simulink model "NavFilterTestHarness24"  (R2024b)
settings: Solver=FixedStepDiscrete  StartTime=startTime  StopTime=endTime  FixedStep=0.001  RelTol=1e-3  EnableMultiTasking=on
undefined symbols (not defined in the file): accel, ADSframe, ADStime, alignTime, angRate, ATTframe, CourseDeg, EAS2TAS, GndSpd, GPSframe, GPStime, Hgt, IMUframe, IMUtime, LatDeg, LngDeg, MagBiasX, MagBiasY, MagBiasZ, MAGframe, MAGtime, MagX, MagY, MagZ, msecHgtDelay, msecMagDelay, msecPosDelay, msecTasDelay, msecVelDelay, Pitch, Roll, Veas, VelD, Yaw
libraries: simulink x9, simulink_need_slupdate x2
(part 2 of 5)

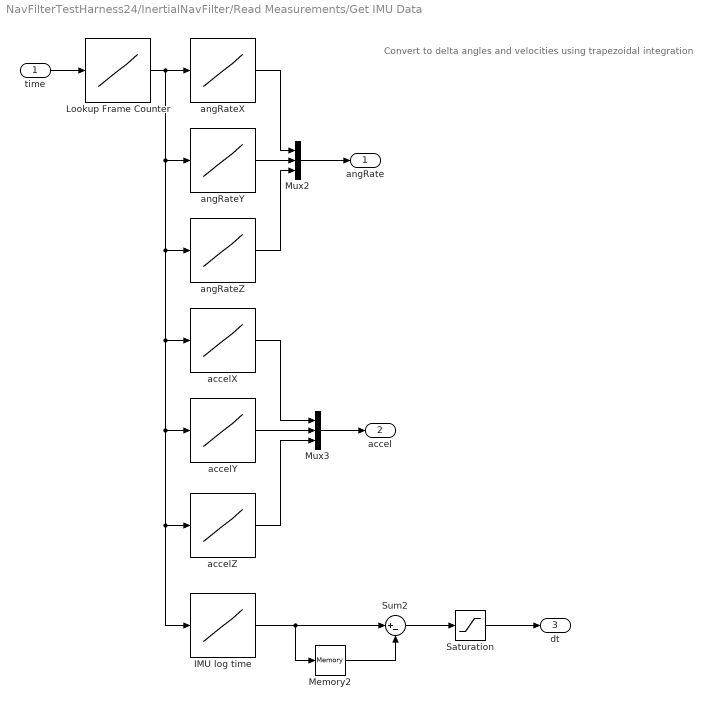
== system NavFilterTestHarness24/InertialNavFilter/Read Measurements/Get IMU Data ==
  note: Convert to delta angles and velocities using trapezoidal integration
  time : Inport
  IMU log time : Lookup_n-D  NumberOfTableDimensions=1  BreakpointsForDimension1=IMUframe  BeginIndexSearchUsingPreviousIndexResult=on  Table=IMUtime  InterpMethod=Flat  DiagnosticForOutOfRangeInput=Error  OutDataTypeStr=single  RndMeth=Simplest
  Lookup Frame Counter : Lookup_n-D  NumberOfTableDimensions=1  BreakpointsForDimension1=IMUtime  BeginIndexSearchUsingPreviousIndexResult=on  Table=IMUframe  InterpMethod=Flat  DiagnosticForOutOfRangeInput=Error  RndMeth=Simplest
  Memory2 : Memory  InheritSampleTime=on
  Mux2 : Mux  Inputs=3
  Mux3 : Mux  Inputs=3
  Saturation : Saturate  UpperLimit=0.04  LowerLimit=0
  Sum2 : Sum  Inputs=|+-  AccumDataTypeStr=single
  accelX : Lookup_n-D  NumberOfTableDimensions=1  BreakpointsForDimension1=IMUframe  BeginIndexSearchUsingPreviousIndexResult=on  Table=accel(:,1)  InterpMethod=Flat  DiagnosticForOutOfRangeInput=Error  OutDataTypeStr=single  RndMeth=Simplest
  accelY : Lookup_n-D  NumberOfTableDimensions=1  BreakpointsForDimension1=IMUframe  BeginIndexSearchUsingPreviousIndexResult=on  Table=accel(:,2)  InterpMethod=Flat  DiagnosticForOutOfRangeInput=Error  OutDataTypeStr=single  RndMeth=Simplest
  accelZ : Lookup_n-D  NumberOfTableDimensions=1  BreakpointsForDimension1=IMUframe  BeginIndexSearchUsingPreviousIndexResult=on  Table=accel(:,3)  InterpMethod=Flat  DiagnosticForOutOfRangeInput=Error  OutDataTypeStr=single  RndMeth=Simplest
  angRateX : Lookup_n-D  NumberOfTableDimensions=1  BreakpointsForDimension1=IMUframe  BeginIndexSearchUsingPreviousIndexResult=on  Table=angRate(:,1)  InterpMethod=Flat  DiagnosticForOutOfRangeInput=Error  OutDataTypeStr=single  RndMeth=Simplest
  angRateY : Lookup_n-D  NumberOfTableDimensions=1  BreakpointsForDimension1=IMUframe  BeginIndexSearchUsingPreviousIndexResult=on  Table=angRate(:,2)  InterpMethod=Flat  DiagnosticForOutOfRangeInput=Error  OutDataTypeStr=single  RndMeth=Simplest
  angRateZ : Lookup_n-D  NumberOfTableDimensions=1  BreakpointsForDimension1=IMUframe  BeginIndexSearchUsingPreviousIndexResult=on  Table=angRate(:,3)  InterpMethod=Flat  DiagnosticForOutOfRangeInput=Error  OutDataTypeStr=single  RndMeth=Simplest
  angRate : Outport  OutDataTypeStr=single
  accel : Outport  Port=2
  dt : Outport  Port=3  OutDataTypeStr=single
  wires:
  accelY/1 -> Mux3/2
  accelX/1 -> Mux3/1
  accelZ/1 -> Mux3/3
  angRateX/1 -> Mux2/1
  angRateY/1 -> Mux2/2
  angRateZ/1 -> Mux2/3
  Lookup Frame Counter/1 -> angRateX/1, angRateY/1, angRateZ/1, accelX/1, accelY/1, accelZ/1, IMU log time/1
  time/1 -> Lookup Frame Counter/1
  IMU log time/1 -> Sum2/1, Memory2/1
  Memory2/1 -> Sum2/2
  Mux2/1 -> angRate/1
  Mux3/1 -> accel/1
  Sum2/1 -> Saturation/1
  Saturation/1 -> dt/1

== system NavFilterTestHarness24/LogData/GetReferenceData/wrapAng to +-pi ==
  In1 : Inport  OutDataTypeStr=single
  If : If  IfExpression=u1 > single(pi)
  If Action Subsystem : Subsystem  TreatAsAtomicUnit=on
  If Action Subsystem1 : Subsystem  TreatAsAtomicUnit=on
  Merge : Merge
  Out1 : Outport  OutDataTypeStr=single
  wires:
  In1/1 -> If Action Subsystem1/1(In1), If Action Subsystem/1(In1), If/1
  If/2 -> If Action Subsystem/Action
  If/1 -> If Action Subsystem1/Action
  If Action Subsystem/1(Out1) -> Merge/1
  If Action Subsystem1/1(Out1) -> Merge/2
  Merge/1 -> Out1/1

== system NavFilterTestHarness24/WatchDog/Get AHRS Data/wrapAng to +-pi ==
  In1 : Inport  OutDataTypeStr=single
  If : If  IfExpression=u1 > single(pi)
  If Action Subsystem : Subsystem  TreatAsAtomicUnit=on
  If Action Subsystem1 : Subsystem  TreatAsAtomicUnit=on
  Merge : Merge
  Out1 : Outport  OutDataTypeStr=single
  wires:
  In1/1 -> If Action Subsystem1/1(In1), If Action Subsystem/1(In1), If/1
  If/2 -> If Action Subsystem/Action
  If/1 -> If Action Subsystem1/Action
  If Action Subsystem/1(Out1) -> Merge/1
  If Action Subsystem1/1(Out1) -> Merge/2
  Merge/1 -> Out1/1

== system NavFilterTestHarness24/InertialNavFilter/CalculateInitialStates/Read AHRS solution/wrapAng to +-pi ==
  In1 : Inport  OutDataTypeStr=single
  If : If  IfExpression=u1 > single(pi)
  If Action Subsystem : Subsystem  TreatAsAtomicUnit=on
  If Action Subsystem1 : Subsystem  TreatAsAtomicUnit=on
  Merge : Merge
  Out1 : Outport  OutDataTypeStr=single
  wires:
  In1/1 -> If Action Subsystem1/1(In1), If Action Subsystem/1(In1), If/1
  If/2 -> If Action Subsystem/Action
  If/1 -> If Action Subsystem1/Action
  If Action Subsystem/1(Out1) -> Merge/1
  If Action Subsystem1/1(Out1) -> Merge/2
  Merge/1 -> Out1/1

== system NavFilterTestHarness24/LogData/GetReferenceData/wrapAng to +-pi/If Action Subsystem ==
  In1 : Inport
  Action Port : ActionPort  ActionPortLabel=else
  Out1 : Outport
  wires:
  In1/1 -> Out1/1

== system NavFilterTestHarness24/LogData/GetReferenceData/wrapAng to +-pi/If Action Subsystem1 ==
  In1 : Inport
  Action Port : ActionPort  ActionPortLabel=if(u1 > single(pi))
  Add : Sum  Inputs=+-
  Constant : Constant  Value=2*pi  OutDataTypeStr=single
  Out1 : Outport
  wires:
  In1/1 -> Add/1
  Add/1 -> Out1/1
  Constant/1 -> Add/2

== system NavFilterTestHarness24/WatchDog/Get AHRS Data/wrapAng to +-pi/If Action Subsystem ==
  In1 : Inport
  Action Port : ActionPort  ActionPortLabel=else
  Out1 : Outport
  wires:
  In1/1 -> Out1/1

== system NavFilterTestHarness24/WatchDog/Get AHRS Data/wrapAng to +-pi/If Action Subsystem1 ==
  In1 : Inport
  Action Port : ActionPort  ActionPortLabel=if(u1 > single(pi))
  Add : Sum  Inputs=+-
  Constant : Constant  Value=2*pi  OutDataTypeStr=single
  Out1 : Outport
  wires:
  In1/1 -> Add/1
  Add/1 -> Out1/1
  Constant/1 -> Add/2

== system NavFilterTestHarness24/InertialNavFilter/CalculateInitialStates/Read AHRS solution/wrapAng to +-pi/If Action Subsystem ==
  In1 : Inport
  Action Port : ActionPort  ActionPortLabel=else
  Out1 : Outport
  wires:
  In1/1 -> Out1/1

== system NavFilterTestHarness24/InertialNavFilter/CalculateInitialStates/Read AHRS solution/wrapAng to +-pi/If Action Subsystem1 ==
  In1 : Inport
  Action Port : ActionPort  ActionPortLabel=if(u1 > single(pi))
  Add : Sum  Inputs=+-
  Constant : Constant  Value=2*pi  OutDataTypeStr=single
  Out1 : Outport
  wires:
  In1/1 -> Add/1
  Add/1 -> Out1/1
  Constant/1 -> Add/2

== matlab function NavFilterTestHarness24/InertialNavFilter/Recall States4 ==
  data: fuseData output; statesStore input; msecStore input; msecDelay input; statesOut output; states input; time input; newDataArrived input
%#codegen
function [fuseData,statesOut]    = RecallStates4(statesStore,msecStore,msecDelay,states,time,newDataArrived)
persistent statesForFusion;
if isempty(statesForFusion)
    statesForFusion = single(zeros(24,1));
end
bestTimeDelta = int32(msecDelay);
bestStoreIndex = 1;
if newDataArrived
    for storeIndex=1:50
        timeDelta = (int32(time*1000) - int32(msecDelay)) - int32(msecStore(storeIndex));
        if (timeDelta < 0)
            timeDelta = -timeDelta;
        end
        if (timeDelta < bestTimeDelta)
            bestStoreIndex = storeIndex;
            bestTimeDelta = timeDelta;
        end
    end
    if (bestTimeDelta < msecDelay) % only output stored state if time accuracy better than just outputtting current states
        for i=1:24
            statesForFusion(i) = statesStore(i,bestStoreIndex);
        end
    else % otherwise output current state
        for i=1:24
            statesForFusion(i) = states(i);
        end
    end
end
statesOut = statesForFusion;
fuseData = newDataArrived;
end

== matlab function NavFilterTestHarness24/InertialNavFilter/Fuse Magnetometer Measurements ==
  data: states input; P input; FuseData input; MagData input; StatesAtMeasTime input; nextStates output; nextP output; innovation output; varInnov output; useCompass input
%#codegen
function [...
    nextStates, ... % state vector after fusion of measurements
    nextP, ... % state covariance matrix after fusion of corrections
    innovation, ... % Magnetometer innovations - milligauss
    varInnov] ... % Innovation variances - millgauss^2
    = FuseMagnetometer( ...
    states, ... % predicted states
    P, ... % predicted covariance
    FuseData, ... % Boolean to initiate fusion of magnetometer measurements
    MagData, ... % Magnetic flux measurements (milliGauss)
    StatesAtMeasTime, ... % states at time of airspeed measurement
    useCompass) % Boolean to indicate that a Magnetometer is being used

persistent q0 q1 q2 q3 magN magE magD;
if isempty(q0)
    q0 = single(1);
end
if isempty(q1)
    q1 = single(0);
end
if isempty(q2)
    q2 = single(0);
end
if isempty(q3)
    q3 = single(0);
end
if isempty(magN)
    magN = single(0);
end
if isempty(magE)
    magE = single(0);
end
if isempty(magD)
    magD = single(0);
end
persistent obsIndex
if isempty(obsIndex)
    obsIndex = 1;
end
persistent SH_MAG
if isempty(SH_MAG)
    SH_MAG = single(zeros(1,9));
end
persistent Tnb
if isempty(Tnb)
    Tnb = single(eye(3,3));
end
persistent MagPred
if isempty(MagPred)
    MagPred = single(zeros(3,1));
end

% declare arrays used to calculate intermediate result in covariance
% and state update
K_MAG = single(zeros(24,1));
H_MAG = single(zeros(1,24));
KH    = single(zeros(24,24));
KHP = single(zeros(24,24));
% define magnetometer measurement error variance (milligauss).
R_MAG = single(50^2);
% declare innovation variances
varInnov = single(zeros(3,1));
% declare innovation vector
innovation = single(zeros(1,3));
% Perform sequential fusion of Magnetometer measurements.
% This assumes that the errors in the dfferent componenets are
% uncorrelated which is not true, however in the absence of covariance
% data fit is the only assumption we can make
% so we might as well take advantage of the computational efficiencies
% associated with sequential fusion
if (useCompass && FuseData) || (useCompass && (obsIndex == 2 || obsIndex == 3))
    % Sequential fusion of XYZ components to spread processing load across
    % three prediction time steps.
    % Calculate observation jacobians and Kalman gains
    if FuseData
        % Copy required states to local variable names
        q0 = StatesAtMeasTime(1);
        q1 = StatesAtMeasTime(2);
        q2 = StatesAtMeasTime(3);
        q3 = StatesAtMeasTime(4);
        magN = StatesAtMeasTime(19);
        magE = StatesAtMeasTime(20);
        magD = StatesAtMeasTime(21);
        % rotate predicted earth components into body axes and calculate
        % predicted measurments
        Tnb = single([q0^2 + q1^2 - q2^2 - q3^2, 2*(q1*q2 + q0*q3) , 2*(q1*q3-q0*q2) ;...
            2*(q1*q2 - q0*q3), q0^2 - q1^2 + q2^2 - q3^2, 2*(q2*q3 + q0*q1);...
            2*(q1*q3 + q0*q2) , 2*(q2*q3 - q0*q1) , q0^2 - q1^2 - q2^2 + q3^2]);
        MagPred = Tnb*StatesAtMeasTime(19:21) + StatesAtMeasTime(22:24);
        % Calculate observation jacobian common terms
        SH_MAG(1) = 2*magD*q3 + 2*magE*q2 + 2*magN*q1;
        SH_MAG(2) = 2*magD*q0 - 2*magE*q1 + 2*magN*q2;
        SH_MAG(3) = 2*magD*q1 + 2*magE*q0 - 2*magN*q3;
        SH_MAG(4) = q3^2;
        SH_MAG(5) = q2^2;
        SH_MAG(6) = q1^2;
        SH_MAG(7) = q0^2;
        SH_MAG(8) = 2*magN*q0;
        SH_MAG(9) = 2*magE*q3;
        % calculate observation jacobian
        H_MAG(1,1) = SH_MAG(8) + SH_MAG(9) - 2*magD*q2;
        H_MAG(1,2) = SH_MAG(1);
        H_MAG(1,3) = 2*magE*q1 - 2*magD*q0 - 2*magN*q2;
        H_MAG(1,4) = SH_MAG(3);
        H_MAG(1,19) = SH_MAG(6) - SH_MAG(5) - SH_MAG(4) + SH_MAG(7);
        H_MAG(1,20) = 2*q0*q3 + 2*q1*q2;
        H_MAG(1,21) = 2*q1*q3 - 2*q0*q2;
        H_MAG(1,22) = 1;
        % calculate Kalman gain
        SK_MX = single(zeros(6,1));
        SK_MX(1) = 1/(P(22,22) + R_MAG + P(2,22)*SH_MAG(1) + P(4,22)*SH_MAG(3) - P(19,22)*(SH_MAG(4) + SH_MAG(5) - SH_MAG(6) - SH_MAG(7)) - (2*magD*q0 - 2*magE*q1 + 2*magN*q2)*(P(22,3) + P(2,3)*SH_MAG(1) + P(4,3)*SH_MAG(3) - P(19,3)*(SH_MAG(4) + SH_MAG(5) - SH_MAG(6) - SH_MAG(7)) + P(20,3)*(2*q0*q3 + 2*q1*q2) - P(21,3)*(2*q0*q2 - 2*q1*q3) - P(3,3)*(2*magD*q0 - 2*magE*q1 + 2*magN*q2) + P(1,3)*(SH_MAG(8) + SH_MAG(9) - 2*magD*q2)) + (SH_MAG(8) + SH_MAG(9) - 2*magD*q2)*(P(22,1) + P(2,1)*SH_MAG(1) + P(4,1)*SH_MAG(3) - P(19,1)*(SH_MAG(4) + SH_MAG(5) - SH_MAG(6) - SH_MAG(7)) + P(20,1)*(2*q0*q3 + 2*q1*q2) - P(21,1)*(2*q0*q2 - 2*q1*q3) - P(3,1)*(2*magD*q0 - 2*magE*q1 + 2*magN*q2) + P(1,1)*(SH_MAG(8) + SH_MAG(9) - 2*magD*q2)) + SH_MAG(1)*(P(22,2) + P(2,2)*SH_MAG(1) + P(4,2)*SH_MAG(3) - P(19,2)*(SH_MAG(4) + SH_MAG(5) - SH_MAG(6) - SH_MAG(7)) + P(20,2)*(2*q0*q3 + 2*q1*q2) - P(21,2)*(2*q0*q2 - 2*q1*q3) - P(3,2)*(2*magD*q0 - 2*magE*q1 + 2*magN*q2) + P(1,2)*(SH_MAG(8) + SH_MAG(9) - 2*magD*q2)) + SH_MAG(3)*(P(22,4) + P(2,4)*SH_MAG(1) + P(4,4)*SH_MAG(3) - P(19,4)*(SH_MAG(4) + SH_MAG(5) - SH_MAG(6) - SH_MAG(7)) + P(20,4)*(2*q0*q3 + 2*q1*q2) - P(21,4)*(2*q0*q2 - 2*q1*q3) - P(3,4)*(2*magD*q0 - 2*magE*q1 + 2*magN*q2) + P(1,4)*(SH_MAG(8) + SH_MAG(9) - 2*magD*q2)) - (SH_MAG(4) + SH_MAG(5) - SH_MAG(6) - SH_MAG(7))*(P(22,19) + P(2,19)*SH_MAG(1) + P(4,19)*SH_MAG(3) - P(19,19)*(SH_MAG(4) + SH_MAG(5) - SH_MAG(6) - SH_MAG(7)) + P(20,19)*(2*q0*q3 + 2*q1*q2) - P(21,19)*(2*q0*q2 - 2*q1*q3) - P(3,19)*(2*magD*q0 - 2*magE*q1 + 2*magN*q2) + P(1,19)*(SH_MAG(8) + SH_MAG(9) - 2*magD*q2)) + P(20,22)*(2*q0*q3 + 2*q1*q2) - P(21,22)*(2*q0*q2 - 2*q1*q3) - P(3,22)*(2*magD*q0 - 2*magE*q1 + 2*magN*q2) + (2*q0*q3 + 2*q1*q2)*(P(22,20) + P(2,20)*SH_MAG(1) + P(4,20)*SH_MAG(3) - P(19,20)*(SH_MAG(4) + SH_MAG(5) - SH_MAG(6) - SH_MAG(7)) + P(20,20)*(2*q0*q3 + 2*q1*q2) - P(21,20)*(2*q0*q2 - 2*q1*q3) - P(3,20)*(2*magD*q0 - 2*magE*q1 + 2*magN*q2) + P(1,20)*(SH_MAG(8) + SH_MAG(9) - 2*magD*q2)) - (2*q0*q2 - 2*q1*q3)*(P(22,21) + P(2,21)*SH_MAG(1) + P(4,21)*SH_MAG(3) - P(19,21)*(SH_MAG(4) + SH_MAG(5) - SH_MAG(6) - SH_MAG(7)) + P(20,21)*(2*q0*q3 + 2*q1*q2) - P(21,21)*(2*q0*q2 - 2*q1*q3) - P(3,21)*(2*magD*q0 - 2*magE*q1 + 2*magN*q2) + P(1,21)*(SH_MAG(8) + SH_MAG(9) - 2*magD*q2)) + P(1,22)*(SH_MAG(8) + SH_MAG(9) - 2*magD*q2));
        SK_MX(2) = SH_MAG(4) + SH_MAG(5) - SH_MAG(6) - SH_MAG(7);
        SK_MX(3) = 2*magD*q0 - 2*magE*q1 + 2*magN*q2;
        SK_MX(4) = SH_MAG(8) + SH_MAG(9) - 2*magD*q2;
        SK_MX(5) = 2*q0*q2 - 2*q1*q3;
        SK_MX(6) = 2*q0*q3 + 2*q1*q2;
        K_MAG(1,1) = SK_MX(1)*(P(1,22) + P(1,2)*SH_MAG(1) + P(1,4)*SH_MAG(3) + P(1,1)*SK_MX(4) - P(1,3)*SK_MX(3) - P(1,19)*SK_MX(2) + P(1,20)*SK_MX(6) - P(1,21)*SK_MX(5));
        K_MAG(2,1) = SK_MX(1)*(P(2,22) + P(2,2)*SH_MAG(1) + P(2,4)*SH_MAG(3) + P(2,1)*SK_MX(4) - P(2,3)*SK_MX(3) - P(2,19)*SK_MX(2) + P(2,20)*SK_MX(6) - P(2,21)*SK_MX(5));
        K_MAG(3,1) = SK_MX(1)*(P(3,22) + P(3,2)*SH_MAG(1) + P(3,4)*SH_MAG(3) + P(3,1)*SK_MX(4) - P(3,3)*SK_MX(3) - P(3,19)*SK_MX(2) + P(3,20)*SK_MX(6) - P(3,21)*SK_MX(5));
        K_MAG(4,1) = SK_MX(1)*(P(4,22) + P(4,2)*SH_MAG(1) + P(4,4)*SH_MAG(3) + P(4,1)*SK_MX(4) - P(4,3)*SK_MX(3) - P(4,19)*SK_MX(2) + P(4,20)*SK_MX(6) - P(4,21)*SK_MX(5));
        K_MAG(5,1) = SK_MX(1)*(P(5,22) + P(5,2)*SH_MAG(1) + P(5,4)*SH_MAG(3) + P(5,1)*SK_MX(4) - P(5,3)*SK_MX(3) - P(5,19)*SK_MX(2) + P(5,20)*SK_MX(6) - P(5,21)*SK_MX(5));
        K_MAG(6,1) = SK_MX(1)*(P(6,22) + P(6,2)*SH_MAG(1) + P(6,4)*SH_MAG(3) + P(6,1)*SK_MX(4) - P(6,3)*SK_MX(3) - P(6,19)*SK_MX(2) + P(6,20)*SK_MX(6) - P(6,21)*SK_MX(5));
        K_MAG(7,1) = SK_MX(1)*(P(7,22) + P(7,2)*SH_MAG(1) + P(7,4)*SH_MAG(3) + P(7,1)*SK_MX(4) - P(7,3)*SK_MX(3) - P(7,19)*SK_MX(2) + P(7,20)*SK_MX(6) - P(7,21)*SK_MX(5));
        K_MAG(8,1) = SK_MX(1)*(P(8,22) + P(8,2)*SH_MAG(1) + P(8,4)*SH_MAG(3) + P(8,1)*SK_MX(4) - P(8,3)*SK_MX(3) - P(8,19)*SK_MX(2) + P(8,20)*SK_MX(6) - P(8,21)*SK_MX(5));
        K_MAG(9,1) = SK_MX(1)*(P(9,22) + P(9,2)*SH_MAG(1) + P(9,4)*SH_MAG(3) + P(9,1)*SK_MX(4) - P(9,3)*SK_MX(3) - P(9,19)*SK_MX(2) + P(9,20)*SK_MX(6) - P(9,21)*SK_MX(5));
        K_MAG(10,1) = SK_MX(1)*(P(10,22) + P(10,2)*SH_MAG(1) + P(10,4)*SH_MAG(3) + P(10,1)*SK_MX(4) - P(10,3)*SK_MX(3) - P(10,19)*SK_MX(2) + P(10,20)*SK_MX(6) - P(10,21)*SK_MX(5));
        K_MAG(11,1) = SK_MX(1)*(P(11,22) + P(11,2)*SH_MAG(1) + P(11,4)*SH_MAG(3) + P(11,1)*SK_MX(4) - P(11,3)*SK_MX(3) - P(11,19)*SK_MX(2) + P(11,20)*SK_MX(6) - P(11,21)*SK_MX(5));
        K_MAG(12,1) = SK_MX(1)*(P(12,22) + P(12,2)*SH_MAG(1) + P(12,4)*SH_MAG(3) + P(12,1)*SK_MX(4) - P(12,3)*SK_MX(3) - P(12,19)*SK_MX(2) + P(12,20)*SK_MX(6) - P(12,21)*SK_MX(5));
        K_MAG(13,1) = SK_MX(1)*(P(13,22) + P(13,2)*SH_MAG(1) + P(13,4)*SH_MAG(3) + P(13,1)*SK_MX(4) - P(13,3)*SK_MX(3) - P(13,19)*SK_MX(2) + P(13,20)*SK_MX(6) - P(13,21)*SK_MX(5));
        K_MAG(14,1) = SK_MX(1)*(P(14,22) + P(14,2)*SH_MAG(1) + P(14,4)*SH_MAG(3) + P(14,1)*SK_MX(4) - P(14,3)*SK_MX(3) - P(14,19)*SK_MX(2) + P(14,20)*SK_MX(6) - P(14,21)*SK_MX(5));
        K_MAG(15,1) = SK_MX(1)*(P(15,22) + P(15,2)*SH_MAG(1) + P(15,4)*SH_MAG(3) + P(15,1)*SK_MX(4) - P(15,3)*SK_MX(3) - P(15,19)*SK_MX(2) + P(15,20)*SK_MX(6) - P(15,21)*SK_MX(5));
        K_MAG(16,1) = SK_MX(1)*(P(16,22) + P(16,2)*SH_MAG(1) + P(16,4)*SH_MAG(3) + P(16,1)*SK_MX(4) - P(16,3)*SK_MX(3) - P(16,19)*SK_MX(2) + P(16,20)*SK_MX(6) - P(16,21)*SK_MX(5));
        K_MAG(17,1) = SK_MX(1)*(P(17,22) + P(17,2)*SH_MAG(1) + P(17,4)*SH_MAG(3) + P(17,1)*SK_MX(4) - P(17,3)*SK_MX(3) - P(17,19)*SK_MX(2) + P(17,20)*SK_MX(6) - P(17,21)*SK_MX(5));
        K_MAG(18,1) = SK_MX(1)*(P(18,22) + P(18,2)*SH_MAG(1) + P(18,4)*SH_MAG(3) + P(18,1)*SK_MX(4) - P(18,3)*SK_MX(3) - P(18,19)*SK_MX(2) + P(18,20)*SK_MX(6) - P(18,21)*SK_MX(5));
        K_MAG(19,1) = SK_MX(1)*(P(19,22) + P(19,2)*SH_MAG(1) + P(19,4)*SH_MAG(3) + P(19,1)*SK_MX(4) - P(19,3)*SK_MX(3) - P(19,19)*SK_MX(2) + P(19,20)*SK_MX(6) - P(19,21)*SK_MX(5));
        K_MAG(20,1) = SK_MX(1)*(P(20,22) + P(20,2)*SH_MAG(1) + P(20,4)*SH_MAG(3) + P(20,1)*SK_MX(4) - P(20,3)*SK_MX(3) - P(20,19)*SK_MX(2) + P(20,20)*SK_MX(6) - P(20,21)*SK_MX(5));
        K_MAG(21,1) = SK_MX(1)*(P(21,22) + P(21,2)*SH_MAG(1) + P(21,4)*SH_MAG(3) + P(21,1)*SK_MX(4) - P(21,3)*SK_MX(3) - P(21,19)*SK_MX(2) + P(21,20)*SK_MX(6) - P(21,21)*SK_MX(5));
        K_MAG(22,1) = SK_MX(1)*(P(22,22) + P(22,2)*SH_MAG(1) + P(22,4)*SH_MAG(3) + P(22,1)*SK_MX(4) - P(22,3)*SK_MX(3) - P(22,19)*SK_MX(2) + P(22,20)*SK_MX(6) - P(22,21)*SK_MX(5));
        K_MAG(23,1) = SK_MX(1)*(P(23,22) + P(23,2)*SH_MAG(1) + P(23,4)*SH_MAG(3) + P(23,1)*SK_MX(4) - P(23,3)*SK_MX(3) - P(23,19)*SK_MX(2) + P(23,20)*SK_MX(6) - P(23,21)*SK_MX(5));
        K_MAG(24,1) = SK_MX(1)*(P(24,22) + P(24,2)*SH_MAG(1) + P(24,4)*SH_MAG(3) + P(24,1)*SK_MX(4) - P(24,3)*SK_MX(3) - P(24,19)*SK_MX(2) + P(24,20)*SK_MX(6) - P(24,21)*SK_MX(5));
        varInnov(1) = 1/SK_MX(1);
        % reset the observation index to 1 (we start by fusing the X
        % measurement)
        obsIndex = 1;
    elseif obsIndex == 2 % we are now fusing the Y measurement
        H_MAG(1,1) = SH_MAG(3);
        H_MAG(1,2) = SH_MAG(2);
        H_MAG(1,3) = SH_MAG(1);
        H_MAG(1,4) = 2*magD*q2 - SH_MAG(9) - SH_MAG(8);
        H_MAG(1,19) = 2*q1*q2 - 2*q0*q3;
        H_MAG(1,20) = SH_MAG(5) - SH_MAG(4) - SH_MAG(6) + SH_MAG(7);
        H_MAG(1,21) = 2*q0*q1 + 2*q2*q3;
        H_MAG(1,23) = 1;
        % calculate the Kalman gain
        SK_MY = single(zeros(5,1));
        SK_MY(1) = 1/(P(23,23) + R_MAG + P(1,23)*SH_MAG(3) + P(2,23)*SH_MAG(2) + P(3,23)*SH_MAG(1) - P(20,23)*(SH_MAG(4) - SH_MAG(5) + SH_MAG(6) - SH_MAG(7)) - (2*q0*q3 - 2*q1*q2)*(P(23,19) + P(1,19)*SH_MAG(3) + P(2,19)*SH_MAG(2) + P(3,19)*SH_MAG(1) - P(20,19)*(SH_MAG(4) - SH_MAG(5) + SH_MAG(6) - SH_MAG(7)) - P(19,19)*(2*q0*q3 - 2*q1*q2) + P(21,19)*(2*q0*q1 + 2*q2*q3) - P(4,19)*(SH_MAG(8) + SH_MAG(9) - 2*magD*q2)) + (2*q0*q1 + 2*q2*q3)*(P(23,21) + P(1,21)*SH_MAG(3) + P(2,21)*SH_MAG(2) + P(3,21)*SH_MAG(1) - P(20,21)*(SH_MAG(4) - SH_MAG(5) + SH_MAG(6) - SH_MAG(7)) - P(19,21)*(2*q0*q3 - 2*q1*q2) + P(21,21)*(2*q0*q1 + 2*q2*q3) - P(4,21)*(SH_MAG(8) + SH_MAG(9) - 2*magD*q2)) - (SH_MAG(8) + SH_MAG(9) - 2*magD*q2)*(P(23,4) + P(1,4)*SH_MAG(3) + P(2,4)*SH_MAG(2) + P(3,4)*SH_MAG(1) - P(20,4)*(SH_MAG(4) - SH_MAG(5) + SH_MAG(6) - SH_MAG(7)) - P(19,4)*(2*q0*q3 - 2*q1*q2) + P(21,4)*(2*q0*q1 + 2*q2*q3) - P(4,4)*(SH_MAG(8) + SH_MAG(9) - 2*magD*q2)) - P(19,23)*(2*q0*q3 - 2*q1*q2) + P(21,23)*(2*q0*q1 + 2*q2*q3) + SH_MAG(3)*(P(23,1) + P(1,1)*SH_MAG(3) + P(2,1)*SH_MAG(2) + P(3,1)*SH_MAG(1) - P(20,1)*(SH_MAG(4) - SH_MAG(5) + SH_MAG(6) - SH_MAG(7)) - P(19,1)*(2*q0*q3 - 2*q1*q2) + P(21,1)*(2*q0*q1 + 2*q2*q3) - P(4,1)*(SH_MAG(8) + SH_MAG(9) - 2*magD*q2)) + SH_MAG(2)*(P(23,2) + P(1,2)*SH_MAG(3) + P(2,2)*SH_MAG(2) + P(3,2)*SH_MAG(1) - P(20,2)*(SH_MAG(4) - SH_MAG(5) + SH_MAG(6) - SH_MAG(7)) - P(19,2)*(2*q0*q3 - 2*q1*q2) + P(21,2)*(2*q0*q1 + 2*q2*q3) - P(4,2)*(SH_MAG(8) + SH_MAG(9) - 2*magD*q2)) + SH_MAG(1)*(P(23,3) + P(1,3)*SH_MAG(3) + P(2,3)*SH_MAG(2) + P(3,3)*SH_MAG(1) - P(20,3)*(SH_MAG(4) - SH_MAG(5) + SH_MAG(6) - SH_MAG(7)) - P(19,3)*(2*q0*q3 - 2*q1*q2) + P(21,3)*(2*q0*q1 + 2*q2*q3) - P(4,3)*(SH_MAG(8) + SH_MAG(9) - 2*magD*q2)) - (SH_MAG(4) - SH_MAG(5) + SH_MAG(6) - SH_MAG(7))*(P(23,20) + P(1,20)*SH_MAG(3) + P(2,20)*SH_MAG(2) + P(3,20)*SH_MAG(1) - P(20,20)*(SH_MAG(4) - SH_MAG(5) + SH_MAG(6) - SH_MAG(7)) - P(19,20)*(2*q0*q3 - 2*q1*q2) + P(21,20)*(2*q0*q1 + 2*q2*q3) - P(4,20)*(SH_MAG(8) + SH_MAG(9) - 2*magD*q2)) - P(4,23)*(SH_MAG(8) + SH_MAG(9) - 2*magD*q2));
        SK_MY(2) = SH_MAG(4) - SH_MAG(5) + SH_MAG(6) - SH_MAG(7);
        SK_MY(3) = SH_MAG(8) + SH_MAG(9) - 2*magD*q2;
        SK_MY(4) = 2*q0*q3 - 2*q1*q2;
        SK_MY(5) = 2*q0*q1 + 2*q2*q3;
        K_MAG(1,1) = SK_MY(1)*(P(1,23) + P(1,1)*SH_MAG(3) + P(1,2)*SH_MAG(2) + P(1,3)*SH_MAG(1) - P(1,4)*SK_MY(3) - P(1,20)*SK_MY(2) - P(1,19)*SK_MY(4) + P(1,21)*SK_MY(5));
        K_MAG(2,1) = SK_MY(1)*(P(2,23) + P(2,1)*SH_MAG(3) + P(2,2)*SH_MAG(2) + P(2,3)*SH_MAG(1) - P(2,4)*SK_MY(3) - P(2,20)*SK_MY(2) - P(2,19)*SK_MY(4) + P(2,21)*SK_MY(5));
        K_MAG(3,1) = SK_MY(1)*(P(3,23) + P(3,1)*SH_MAG(3) + P(3,2)*SH_MAG(2) + P(3,3)*SH_MAG(1) - P(3,4)*SK_MY(3) - P(3,20)*SK_MY(2) - P(3,19)*SK_MY(4) + P(3,21)*SK_MY(5));
        K_MAG(4,1) = SK_MY(1)*(P(4,23) + P(4,1)*SH_MAG(3) + P(4,2)*SH_MAG(2) + P(4,3)*SH_MAG(1) - P(4,4)*SK_MY(3) - P(4,20)*SK_MY(2) - P(4,19)*SK_MY(4) + P(4,21)*SK_MY(5));
        K_MAG(5,1) = SK_MY(1)*(P(5,23) + P(5,1)*SH_MAG(3) + P(5,2)*SH_MAG(2) + P(5,3)*SH_MAG(1) - P(5,4)*SK_MY(3) - P(5,20)*SK_MY(2) - P(5,19)*SK_MY(4) + P(5,21)*SK_MY(5));
        K_MAG(6,1) = SK_MY(1)*(P(6,23) + P(6,1)*SH_MAG(3) + P(6,2)*SH_MAG(2) + P(6,3)*SH_MAG(1) - P(6,4)*SK_MY(3) - P(6,20)*SK_MY(2) - P(6,19)*SK_MY(4) + P(6,21)*SK_MY(5));
        K_MAG(7,1) = SK_MY(1)*(P(7,23) + P(7,1)*SH_MAG(3) + P(7,2)*SH_MAG(2) + P(7,3)*SH_MAG(1) - P(7,4)*SK_MY(3) - P(7,20)*SK_MY(2) - P(7,19)*SK_MY(4) + P(7,21)*SK_MY(5));
        K_MAG(8,1) = SK_MY(1)*(P(8,23) + P(8,1)*SH_MAG(3) + P(8,2)*SH_MAG(2) + P(8,3)*SH_MAG(1) - P(8,4)*SK_MY(3) - P(8,20)*SK_MY(2) - P(8,19)*SK_MY(4) + P(8,21)*SK_MY(5));
        K_MAG(9,1) = SK_MY(1)*(P(9,23) + P(9,1)*SH_MAG(3) + P(9,2)*SH_MAG(2) + P(9,3)*SH_MAG(1) - P(9,4)*SK_MY(3) - P(9,20)*SK_MY(2) - P(9,19)*SK_MY(4) + P(9,21)*SK_MY(5));
        K_MAG(10,1) = SK_MY(1)*(P(10,23) + P(10,1)*SH_MAG(3) + P(10,2)*SH_MAG(2) + P(10,3)*SH_MAG(1) - P(10,4)*SK_MY(3) - P(10,20)*SK_MY(2) - P(10,19)*SK_MY(4) + P(10,21)*SK_MY(5));
        K_MAG(11,1) = SK_MY(1)*(P(11,23) + P(11,1)*SH_MAG(3) + P(11,2)*SH_MAG(2) + P(11,3)*SH_MAG(1) - P(11,4)*SK_MY(3) - P(11,20)*SK_MY(2) - P(11,19)*SK_MY(4) + P(11,21)*SK_MY(5));
        K_MAG(12,1) = SK_MY(1)*(P(12,23) + P(12,1)*SH_MAG(3) + P(12,2)*SH_MAG(2) + P(12,3)*SH_MAG(1) - P(12,4)*SK_MY(3) - P(12,20)*SK_MY(2) - P(12,19)*SK_MY(4) + P(12,21)*SK_MY(5));
        K_MAG(13,1) = SK_MY(1)*(P(13,23) + P(13,1)*SH_MAG(3) + P(13,2)*SH_MAG(2) + P(13,3)*SH_MAG(1) - P(13,4)*SK_MY(3) - P(13,20)*SK_MY(2) - P(13,19)*SK_MY(4) + P(13,21)*SK_MY(5));
        K_MAG(14,1) = SK_MY(1)*(P(14,23) + P(14,1)*SH_MAG(3) + P(14,2)*SH_MAG(2) + P(14,3)*SH_MAG(1) - P(14,4)*SK_MY(3) - P(14,20)*SK_MY(2) - P(14,19)*SK_MY(4) + P(14,21)*SK_MY(5));
        K_MAG(15,1) = SK_MY(1)*(P(15,23) + P(15,1)*SH_MAG(3) + P(15,2)*SH_MAG(2) + P(15,3)*SH_MAG(1) - P(15,4)*SK_MY(3) - P(15,20)*SK_MY(2) - P(15,19)*SK_MY(4) + P(15,21)*SK_MY(5));
        K_MAG(16,1) = SK_MY(1)*(P(16,23) + P(16,1)*SH_MAG(3) + P(16,2)*SH_MAG(2) + P(16,3)*SH_MAG(1) - P(16,4)*SK_MY(3) - P(16,20)*SK_MY(2) - P(16,19)*SK_MY(4) + P(16,21)*SK_MY(5));
        K_MAG(17,1) = SK_MY(1)*(P(17,23) + P(17,1)*SH_MAG(3) + P(17,2)*SH_MAG(2) + P(17,3)*SH_MAG(1) - P(17,4)*SK_MY(3) - P(17,20)*SK_MY(2) - P(17,19)*SK_MY(4) + P(17,21)*SK_MY(5));
        K_MAG(18,1) = SK_MY(1)*(P(18,23) + P(18,1)*SH_MAG(3) + P(18,2)*SH_MAG(2) + P(18,3)*SH_MAG(1) - P(18,4)*SK_MY(3) - P(18,20)*SK_MY(2) - P(18,19)*SK_MY(4) + P(18,21)*SK_MY(5));
        K_MAG(19,1) = SK_MY(1)*(P(19,23) + P(19,1)*SH_MAG(3) + P(19,2)*SH_MAG(2) + P(19,3)*SH_MAG(1) - P(19,4)*SK_MY(3) - P(19,20)*SK_MY(2) - P(19,19)*SK_MY(4) + P(19,21)*SK_MY(5));
        K_MAG(20,1) = SK_MY(1)*(P(20,23) + P(20,1)*SH_MAG(3) + P(20,2)*SH_MAG(2) + P(20,3)*SH_MAG(1) - P(20,4)*SK_MY(3) - P(20,20)*SK_MY(2) - P(20,19)*SK_MY(4) + P(20,21)*SK_MY(5));
        K_MAG(21,1) = SK_MY(1)*(P(21,23) + P(21,1)*SH_MAG(3) + P(21,2)*SH_MAG(2) + P(21,3)*SH_MAG(1) - P(21,4)*SK_MY(3) - P(21,20)*SK_MY(2) - P(21,19)*SK_MY(4) + P(21,21)*SK_MY(5));
        K_MAG(22,1) = SK_MY(1)*(P(22,23) + P(22,1)*SH_MAG(3) + P(22,2)*SH_MAG(2) + P(22,3)*SH_MAG(1) - P(22,4)*SK_MY(3) - P(22,20)*SK_MY(2) - P(22,19)*SK_MY(4) + P(22,21)*SK_MY(5));
        K_MAG(23,1) = SK_MY(1)*(P(23,23) + P(23,1)*SH_MAG(3) + P(23,2)*SH_MAG(2) + P(23,3)*SH_MAG(1) - P(23,4)*SK_MY(3) - P(23,20)*SK_MY(2) - P(23,19)*SK_MY(4) + P(23,21)*SK_MY(5));
        K_MAG(24,1) = SK_MY(1)*(P(24,23) + P(24,1)*SH_MAG(3) + P(24,2)*SH_MAG(2) + P(24,3)*SH_MAG(1) - P(24,4)*SK_MY(3) - P(24,20)*SK_MY(2) - P(24,19)*SK_MY(4) + P(24,21)*SK_MY(5));
        varInnov(2) = 1/SK_MY(1);
    elseif obsIndex == 3 % we ar now fusing the Z measurement
        % calculate the observation jacobian
        H_MAG(1,1) = SH_MAG(2);
        H_MAG(1,2) = 2*magN*q3 - 2*magE*q0 - 2*magD*q1;
        H_MAG(1,3) = SH_MAG(8) + SH_MAG(9) - 2*magD*q2;
        H_MAG(1,4) = SH_MAG(1);
        H_MAG(1,19) = 2*q0*q2 + 2*q1*q3;
        H_MAG(1,20) = 2*q2*q3 - 2*q0*q1;
        H_MAG(1,21) = SH_MAG(4) - SH_MAG(5) - SH_MAG(6) + SH_MAG(7);
        H_MAG(1,24) = 1;
        % calculate the Kalman gain
        SK_MZ = single(zeros(6,1));
        SK_MZ(1) = 1/(P(24,24) + R_MAG + P(1,24)*SH_MAG(2) + P(4,24)*SH_MAG(1) + P(21,24)*(SH_MAG(4) - SH_MAG(5) - SH_MAG(6) + SH_MAG(7)) - (2*magD*q1 + 2*magE*q0 - 2*magN*q3)*(P(24,2) + P(1,2)*SH_MAG(2) + P(4,2)*SH_MAG(1) + P(21,2)*(SH_MAG(4) - SH_MAG(5) - SH_MAG(6) + SH_MAG(7)) + P(19,2)*(2*q0*q2 + 2*q1*q3) - P(20,2)*(2*q0*q1 - 2*q2*q3) - P(2,2)*(2*magD*q1 + 2*magE*q0 - 2*magN*q3) + P(3,2)*(SH_MAG(8) + SH_MAG(9) - 2*magD*q2)) + (SH_MAG(8) + SH_MAG(9) - 2*magD*q2)*(P(24,3) + P(1,3)*SH_MAG(2) + P(4,3)*SH_MAG(1) + P(21,3)*(SH_MAG(4) - SH_MAG(5) - SH_MAG(6) + SH_MAG(7)) + P(19,3)*(2*q0*q2 + 2*q1*q3) - P(20,3)*(2*q0*q1 - 2*q2*q3) - P(2,3)*(2*magD*q1 + 2*magE*q0 - 2*magN*q3) + P(3,3)*(SH_MAG(8) + SH_MAG(9) - 2*magD*q2)) + SH_MAG(2)*(P(24,1) + P(1,1)*SH_MAG(2) + P(4,1)*SH_MAG(1) + P(21,1)*(SH_MAG(4) - SH_MAG(5) - SH_MAG(6) + SH_MAG(7)) + P(19,1)*(2*q0*q2 + 2*q1*q3) - P(20,1)*(2*q0*q1 - 2*q2*q3) - P(2,1)*(2*magD*q1 + 2*magE*q0 - 2*magN*q3) + P(3,1)*(SH_MAG(8) + SH_MAG(9) - 2*magD*q2)) + SH_MAG(1)*(P(24,4) + P(1,4)*SH_MAG(2) + P(4,4)*SH_MAG(1) + P(21,4)*(SH_MAG(4) - SH_MAG(5) - SH_MAG(6) + SH_MAG(7)) + P(19,4)*(2*q0*q2 + 2*q1*q3) - P(20,4)*(2*q0*q1 - 2*q2*q3) - P(2,4)*(2*magD*q1 + 2*magE*q0 - 2*magN*q3) + P(3,4)*(SH_MAG(8) + SH_MAG(9) - 2*magD*q2)) + (SH_MAG(4) - SH_MAG(5) - SH_MAG(6) + SH_MAG(7))*(P(24,21) + P(1,21)*SH_MAG(2) + P(4,21)*SH_MAG(1) + P(21,21)*(SH_MAG(4) - SH_MAG(5) - SH_MAG(6) + SH_MAG(7)) + P(19,21)*(2*q0*q2 + 2*q1*q3) - P(20,21)*(2*q0*q1 - 2*q2*q3) - P(2,21)*(2*magD*q1 + 2*magE*q0 - 2*magN*q3) + P(3,21)*(SH_MAG(8) + SH_MAG(9) - 2*magD*q2)) + P(19,24)*(2*q0*q2 + 2*q1*q3) - P(20,24)*(2*q0*q1 - 2*q2*q3) - P(2,24)*(2*magD*q1 + 2*magE*q0 - 2*magN*q3) + (2*q0*q2 + 2*q1*q3)*(P(24,19) + P(1,19)*SH_MAG(2) + P(4,19)*SH_MAG(1) + P(21,19)*(SH_MAG(4) - SH_MAG(5) - SH_MAG(6) + SH_MAG(7)) + P(19,19)*(2*q0*q2 + 2*q1*q3) - P(20,19)*(2*q0*q1 - 2*q2*q3) - P(2,19)*(2*magD*q1 + 2*magE*q0 - 2*magN*q3) + P(3,19)*(SH_MAG(8) + SH_MAG(9) - 2*magD*q2)) - (2*q0*q1 - 2*q2*q3)*(P(24,20) + P(1,20)*SH_MAG(2) + P(4,20)*SH_MAG(1) + P(21,20)*(SH_MAG(4) - SH_MAG(5) - SH_MAG(6) + SH_MAG(7)) + P(19,20)*(2*q0*q2 + 2*q1*q3) - P(20,20)*(2*q0*q1 - 2*q2*q3) - P(2,20)*(2*magD*q1 + 2*magE*q0 - 2*magN*q3) + P(3,20)*(SH_MAG(8) + SH_MAG(9) - 2*magD*q2)) + P(3,24)*(SH_MAG(8) + SH_MAG(9) - 2*magD*q2));
        SK_MZ(2) = SH_MAG(4) - SH_MAG(5) - SH_MAG(6) + SH_MAG(7);
        SK_MZ(3) = 2*magD*q1 + 2*magE*q0 - 2*magN*q3;
        SK_MZ(4) = SH_MAG(8) + SH_MAG(9) - 2*magD*q2;
        SK_MZ(5) = 2*q0*q1 - 2*q2*q3;
        SK_MZ(6) = 2*q0*q2 + 2*q1*q3;
        K_MAG(1,1) = SK_MZ(1)*(P(1,24) + P(1,1)*SH_MAG(2) + P(1,4)*SH_MAG(1) - P(1,2)*SK_MZ(3) + P(1,3)*SK_MZ(4) + P(1,21)*SK_MZ(2) + P(1,19)*SK_MZ(6) - P(1,20)*SK_MZ(5));
        K_MAG(2,1) = SK_MZ(1)*(P(2,24) + P(2,1)*SH_MAG(2) + P(2,4)*SH_MAG(1) - P(2,2)*SK_MZ(3) + P(2,3)*SK_MZ(4) + P(2,21)*SK_MZ(2) + P(2,19)*SK_MZ(6) - P(2,20)*SK_MZ(5));
        K_MAG(3,1) = SK_MZ(1)*(P(3,24) + P(3,1)*SH_MAG(2) + P(3,4)*SH_MAG(1) - P(3,2)*SK_MZ(3) + P(3,3)*SK_MZ(4) + P(3,21)*SK_MZ(2) + P(3,19)*SK_MZ(6) - P(3,20)*SK_MZ(5));
        K_MAG(4,1) = SK_MZ(1)*(P(4,24) + P(4,1)*SH_MAG(2) + P(4,4)*SH_MAG(1) - P(4,2)*SK_MZ(3) + P(4,3)*SK_MZ(4) + P(4,21)*SK_MZ(2) + P(4,19)*SK_MZ(6) - P(4,20)*SK_MZ(5));
        K_MAG(5,1) = SK_MZ(1)*(P(5,24) + P(5,1)*SH_MAG(2) + P(5,4)*SH_MAG(1) - P(5,2)*SK_MZ(3) + P(5,3)*SK_MZ(4) + P(5,21)*SK_MZ(2) + P(5,19)*SK_MZ(6) - P(5,20)*SK_MZ(5));
        K_MAG(6,1) = SK_MZ(1)*(P(6,24) + P(6,1)*SH_MAG(2) + P(6,4)*SH_MAG(1) - P(6,2)*SK_MZ(3) + P(6,3)*SK_MZ(4) + P(6,21)*SK_MZ(2) + P(6,19)*SK_MZ(6) - P(6,20)*SK_MZ(5));
        K_MAG(7,1) = SK_MZ(1)*(P(7,24) + P(7,1)*SH_MAG(2) + P(7,4)*SH_MAG(1) - P(7,2)*SK_MZ(3) + P(7,3)*SK_MZ(4) + P(7,21)*SK_MZ(2) + P(7,19)*SK_MZ(6) - P(7,20)*SK_MZ(5));
        K_MAG(8,1) = SK_MZ(1)*(P(8,24) + P(8,1)*SH_MAG(2) + P(8,4)*SH_MAG(1) - P(8,2)*SK_MZ(3) + P(8,3)*SK_MZ(4) + P(8,21)*SK_MZ(2) + P(8,19)*SK_MZ(6) - P(8,20)*SK_MZ(5));
        K_MAG(9,1) = SK_MZ(1)*(P(9,24) + P(9,1)*SH_MAG(2) + P(9,4)*SH_MAG(1) - P(9,2)*SK_MZ(3) + P(9,3)*SK_MZ(4) + P(9,21)*SK_MZ(2) + P(9,19)*SK_MZ(6) - P(9,20)*SK_MZ(5));
        K_MAG(10,1) = SK_MZ(1)*(P(10,24) + P(10,1)*SH_MAG(2) + P(10,4)*SH_MAG(1) - P(10,2)*SK_MZ(3) + P(10,3)*SK_MZ(4) + P(10,21)*SK_MZ(2) + P(10,19)*SK_MZ(6) - P(10,20)*SK_MZ(5));
        K_MAG(11,1) = SK_MZ(1)*(P(11,24) + P(11,1)*SH_MAG(2) + P(11,4)*SH_MAG(1) - P(11,2)*SK_MZ(3) + P(11,3)*SK_MZ(4) + P(11,21)*SK_MZ(2) + P(11,19)*SK_MZ(6) - P(11,20)*SK_MZ(5));
        K_MAG(12,1) = SK_MZ(1)*(P(12,24) + P(12,1)*SH_MAG(2) + P(12,4)*SH_MAG(1) - P(12,2)*SK_MZ(3) + P(12,3)*SK_MZ(4) + P(12,21)*SK_MZ(2) + P(12,19)*SK_MZ(6) - P(12,20)*SK_MZ(5));
        K_MAG(13,1) = SK_MZ(1)*(P(13,24) + P(13,1)*SH_MAG(2) + P(13,4)*SH_MAG(1) - P(13,2)*SK_MZ(3) + P(13,3)*SK_MZ(4) + P(13,21)*SK_MZ(2) + P(13,19)*SK_MZ(6) - P(13,20)*SK_MZ(5));
        K_MAG(14,1) = SK_MZ(1)*(P(14,24) + P(14,1)*SH_MAG(2) + P(14,4)*SH_MAG(1) - P(14,2)*SK_MZ(3) + P(14,3)*SK_MZ(4) + P(14,21)*SK_MZ(2) + P(14,19)*SK_MZ(6) - P(14,20)*SK_MZ(5));
        K_MAG(15,1) = SK_MZ(1)*(P(15,24) + P(15,1)*SH_MAG(2) + P(15,4)*SH_MAG(1) - P(15,2)*SK_MZ(3) + P(15,3)*SK_MZ(4) + P(15,21)*SK_MZ(2) + P(15,19)*SK_MZ(6) - P(15,20)*SK_MZ(5));
        K_MAG(16,1) = SK_MZ(1)*(P(16,24) + P(16,1)*SH_MAG(2) + P(16,4)*SH_MAG(1) - P(16,2)*SK_MZ(3) + P(16,3)*SK_MZ(4) + P(16,21)*SK_MZ(2) + P(16,19)*SK_MZ(6) - P(16,20)*SK_MZ(5));
        K_MAG(17,1) = SK_MZ(1)*(P(17,24) + P(17,1)*SH_MAG(2) + P(17,4)*SH_MAG(1) - P(17,2)*SK_MZ(3) + P(17,3)*SK_MZ(4) + P(17,21)*SK_MZ(2) + P(17,19)*SK_MZ(6) - P(17,20)*SK_MZ(5));
        K_MAG(18,1) = SK_MZ(1)*(P(18,24) + P(18,1)*SH_MAG(2) + P(18,4)*SH_MAG(1) - P(18,2)*SK_MZ(3) + P(18,3)*SK_MZ(4) + P(18,21)*SK_MZ(2) + P(18,19)*SK_MZ(6) - P(18,20)*SK_MZ(5));
        K_MAG(19,1) = SK_MZ(1)*(P(19,24) + P(19,1)*SH_MAG(2) + P(19,4)*SH_MAG(1) - P(19,2)*SK_MZ(3) + P(19,3)*SK_MZ(4) + P(19,21)*SK_MZ(2) + P(19,19)*SK_MZ(6) - P(19,20)*SK_MZ(5));
        K_MAG(20,1) = SK_MZ(1)*(P(20,24) + P(20,1)*SH_MAG(2) + P(20,4)*SH_MAG(1) - P(20,2)*SK_MZ(3) + P(20,3)*SK_MZ(4) + P(20,21)*SK_MZ(2) + P(20,19)*SK_MZ(6) - P(20,20)*SK_MZ(5));
        K_MAG(21,1) = SK_MZ(1)*(P(21,24) + P(21,1)*SH_MAG(2) + P(21,4)*SH_MAG(1) - P(21,2)*SK_MZ(3) + P(21,3)*SK_MZ(4) + P(21,21)*SK_MZ(2) + P(21,19)*SK_MZ(6) - P(21,20)*SK_MZ(5));
        K_MAG(22,1) = SK_MZ(1)*(P(22,24) + P(22,1)*SH_MAG(2) + P(22,4)*SH_MAG(1) - P(22,2)*SK_MZ(3) + P(22,3)*SK_MZ(4) + P(22,21)*SK_MZ(2) + P(22,19)*SK_MZ(6) - P(22,20)*SK_MZ(5));
        K_MAG(23,1) = SK_MZ(1)*(P(23,24) + P(23,1)*SH_MAG(2) + P(23,4)*SH_MAG(1) - P(23,2)*SK_MZ(3) + P(23,3)*SK_MZ(4) + P(23,21)*SK_MZ(2) + P(23,19)*SK_MZ(6) - P(23,20)*SK_MZ(5));
        K_MAG(24,1) = SK_MZ(1)*(P(24,24) + P(24,1)*SH_MAG(2) + P(24,4)*SH_MAG(1) - P(24,2)*SK_MZ(3) + P(24,3)*SK_MZ(4) + P(24,21)*SK_MZ(2) + P(24,19)*SK_MZ(6) - P(24,20)*SK_MZ(5));
        varInnov(3) = 1/SK_MZ(1);
    end
    % Calculate the measurement innovation
    innovation(obsIndex) = MagPred(obsIndex) - MagData(obsIndex);
    % Check the innovation for consistencey and don't fuse if > 5Sigma
    if ((innovation(obsIndex)^2) / varInnov(obsIndex)) < 25.0
        xk = K_MAG * innovation(obsIndex);
        states = states - xk;
        % normalise the quaternion states
        quatMag = sqrt(states(1)^2 + states(2)^2 + states(3)^2 + states(4)^2);
        if (quatMag > 1e-12)
            states(1:4) = states(1:4) / quatMag;
        end
        % correct the covariance P = (I - K*H)*P
        % take advantage of the empty columns in KH to reduce the
        % number of operations
        for i = 1:24
            for j = 1:4
                KH(i,j) = K_MAG(i,1)*H_MAG(1,j);
            end
            for j = 19:24
                KH(i,j) = K_MAG(i,1)*H_MAG(1,j);
            end
        end
        for i = 1:24
            for j = 1:24
                for k = 1:4
                    KHP(i,j) = KHP(i,j) + KH(i,k)*P(k,j);
                end
                for k = 19:24
                    KHP(i,j) = KHP(i,j) + KH(i,k)*P(k,j);
                end
            end
        end
        P = P - KHP;
    end
    % increment observation index
    obsIndex = obsIndex + 1;
end
% Set output for states and covariance
nextP = P;
nextStates = states;
end

== matlab function NavFilterTestHarness24/LogData/Embedded MATLAB Function ==
  data: eulVar output; states input; quatCov input
%#codegen
function eulVar  = calcEulerVariances(states,quatCov)

eulVar = zeros(1,3);

q0 = states(1);
q1 = states(2);
q2 = states(3);
q3 = states(4);

SJ = zeros(5,1);
SJ(1) = 1/(((2*q0*q3 + 2*q1*q2)/q0^2 + q1^2 - q2^2 - q3^2)^2 + 1);
SJ(2) = 1/(((2*q0*q1 + 2*q2*q3)/q0^2 - q1^2 - q2^2 + q3^2)^2 + 1);
SJ(3) = 1/(1 - (2*q0*q2 - 2*q1*q3)^2)^(1/2);
SJ(4) = 1/q0^2;
SJ(5) = 1/q0^3;

J = zeros(3,4);
J(1,1) = SJ(2)*(2*q1*SJ(4) - 2*SJ(5)*(2*q0*q1 + 2*q2*q3));
J(1,2) = -SJ(2)*(2*q1 - 2/q0);
J(1,3) = -SJ(2)*(2*q2 - 2*q3*SJ(4));
J(1,4) = SJ(2)*(2*q3 + 2*q2*SJ(4));
J(2,1) = 2*q2*SJ(3);
J(2,2) = -2*q3*SJ(3);
J(2,3) = 2*q0*SJ(3);
J(2,4) = -2*q1*SJ(3);
J(3,1) = SJ(1)*(2*q3*SJ(4) - 2*SJ(5)*(2*q0*q3 + 2*q1*q2));
J(3,2) = SJ(1)*(2*q1 + 2*q2*SJ(4));
J(3,3) = -SJ(1)*(2*q2 - 2*q1*SJ(4));
J(3,4) = -SJ(1)*(2*q3 - 2/q0);

% Transform the Euler angle covariances into the equivalent quaternion covariances
eulCov = J*quatCov*transpose(J);

eulVar(1) = eulCov(1,1);
eulVar(2) = eulCov(2,2);
eulVar(3) = eulCov(3,3);


return

== matlab function NavFilterTestHarness24/LogData/Convert GPS Data ==
  data: LatLongDeg input; GndSpd input; CourseDeg input; VelD input; VelNED output; PosNE output; RefLatLongDeg input
%#codegen
function [VelNED,PosNE]   = ConvertGpsData(LatLongDeg,GndSpd,CourseDeg,VelD,RefLatLongDeg)

% Do a conversion from lat,long to local North.Est position relative to a
% reference point using WGS-84 eaerth radius and using a simple spherical
% earth model
% Convert GPS course and speed to North and East velocity components

deg2rad = single(pi/180);
earthRadius = single(6378145);

PosNE = single(zeros(2,1));
VelNED = single(zeros(3,1));
LatLongDelta = (LatLongDeg-RefLatLongDeg) * deg2rad;
PosNE(1) = earthRadius * LatLongDelta(1);
PosNE(2) = earthRadius * cos(RefLatLongDeg(1)*deg2rad) * LatLongDelta(2);
VelNED(1) = GndSpd*cos(CourseDeg*deg2rad);
VelNED(2) = GndSpd*sin(CourseDeg*deg2rad);
VelNED(3) = VelD;

return

== matlab function NavFilterTestHarness24/InertialNavFilter/Recall States5 ==
  data: fuseData output; statesStore input; msecStore input; msecDelay input; statesOut output; states input; time input; newDataArrived input
%#codegen
function [fuseData,statesOut]    = RecallStates5(statesStore,msecStore,msecDelay,states,time,newDataArrived)
persistent statesForFusion;
if isempty(statesForFusion)
    statesForFusion = single(zeros(24,1));
end
bestTimeDelta = int32(msecDelay);
bestStoreIndex = 1;
if newDataArrived
    for storeIndex=1:50
        timeDelta = (int32(time*1000) - int32(msecDelay)) - int32(msecStore(storeIndex));
        if (timeDelta < 0)
            timeDelta = -timeDelta;
        end
        if (timeDelta < bestTimeDelta)
            bestStoreIndex = storeIndex;
            bestTimeDelta = timeDelta;
        end
    end
    if (bestTimeDelta < msecDelay) % only output stored state if time accuracy better than just outputtting current states
        for i=1:24
            statesForFusion(i) = statesStore(i,bestStoreIndex);
        end
    else % otherwise output current state
        for i=1:24
            statesForFusion(i) = states(i);
        end
    end
end
statesOut = statesForFusion;
fuseData = newDataArrived;
end

== matlab function NavFilterTestHarness24/InertialNavFilter/Read Measurements/Convert GPS Data ==
  data: VelNED output; PosNE output; GPS_DataArrived input; RefLatLongDeg input; LatLongDeg input; GndSpd input; CourseDeg input; VelD input
%#codegen
function [VelNED,PosNE]   = ConvertGpsData(GPS_DataArrived,RefLatLongDeg,LatLongDeg,GndSpd,CourseDeg,VelD)

% Do a conversion from lat,long to local North.Est position relative to a
% reference point using WGS-84 eaerth radius and using a simple spherical
% earth model
% Convert GPS course and speed to North and East velocity components

deg2rad = single(pi/180);
earthRadius = single(6378145);

PosNE = single(zeros(2,1));
VelNED = single(zeros(3,1));
LatLongDelta = (LatLongDeg-RefLatLongDeg) * deg2rad;
PosNE(1) = earthRadius * LatLongDelta(1);
PosNE(2) = earthRadius * cos(RefLatLongDeg(1)*deg2rad) * LatLongDelta(2);
VelNED(1) = GndSpd*cos(CourseDeg*deg2rad);
VelNED(2) = GndSpd*sin(CourseDeg*deg2rad);
VelNED(3) = VelD;

return

== matlab function NavFilterTestHarness24/InertialNavFilter/Read Measurements/Calculate Delta Angles & Velocities ==
  data: delAngIMU output; delVelIMU output; angRateIMU input; accelIMU input; dtIMU input
%#codegen
function [delAngIMU,delVelIMU]  = CalcDeltaAngVel(angRateIMU, accelIMU, dtIMU)

persistent prevAngRateIMU;
if isempty(prevAngRateIMU)
    prevAngRateIMU = single([0;0;0]);
end
persistent prevAccelIMU;
if isempty(prevAccelIMU)
    prevAccelIMU = single([0;0;0]);
end

% Apply trapezoidal integration
delAngIMU = 0.5*dtIMU*(angRateIMU + prevAngRateIMU);
delVelIMU = 0.5*dtIMU*(accelIMU   + prevAccelIMU  );

prevAngRateIMU = angRateIMU;
prevAccelIMU   = accelIMU;

end

== matlab function NavFilterTestHarness24/InertialNavFilter/Store States ==
  data: states input; time input; statesStoreOut output; msecStoreOut output
%#codegen
function [statesStoreOut,msecStoreOut]   = StoreStates(states,time)


persistent statesStore;
if isempty(statesStore)
    statesStore = single(zeros(24,50));
end

persistent index;
if isempty(index)
    index = 1;
end

persistent msecStore;
if isempty(msecStore)
    msecStore = uint32(zeros(1,50));
end

if (index > 50)
    index = 1;
end
for i=1:24
    statesStore(i,index) = states(i);
end
msecStore(index) = round(time*1000);
index = index + 1;

statesStoreOut = statesStore;
msecStoreOut =  msecStore;

end

== matlab function NavFilterTestHarness24/InertialNavFilter/Recall States1 ==
  data: fuseData output; statesStore input; msecStore input; msecDelay input; statesOut output; states input; time input; newDataArrived input
%#codegen
function [fuseData,statesOut]    = RecallStates1(statesStore,msecStore,msecDelay,states,time,newDataArrived)
persistent statesForFusion;
if isempty(statesForFusion)
    statesForFusion = single(zeros(24,1));
end
bestTimeDelta = int32(msecDelay);
bestStoreIndex = 1;
if newDataArrived
    for storeIndex=1:50
        timeDelta = (int32(time*1000) - int32(msecDelay)) - int32(msecStore(storeIndex));
        if (timeDelta < 0)
            timeDelta = -timeDelta;
        end
        if (timeDelta < bestTimeDelta)
            bestStoreIndex = storeIndex;
            bestTimeDelta = timeDelta;
        end
    end
    if (bestTimeDelta < msecDelay) % only output stored state if time accuracy better than just outputtting current states
        for i=1:24
            statesForFusion(i) = statesStore(i,bestStoreIndex);
        end
    else % otherwise output current state
        for i=1:24
            statesForFusion(i) = states(i);
        end
    end
end
statesOut = statesForFusion;
fuseData = newDataArrived;
end

== matlab function NavFilterTestHarness24/InertialNavFilter/Fuse Vel Pos Measurements ==
  data: states input; P input; accNavMag input; FuseVelData input; VelNED input; StatesAtVelTime input; FusePosData input; PosNE input; StatesAtPosTime input; FuseHgtData input; HgtMea input; nextStates output; nextP output; innovation output; varInnov output; StatesAtHgtTime input; useAirspeed input
%#codegen
function [...
    nextStates, ... % state vector after fusion of measurements (q0, ... , q3, VelN,E,D, PosN,E,D, WindN,E, P0, camera roll pitch yaw misalignment)
    nextP, ... % state covariance matrix after fusion of corrections
    innovation,... % NED velocity and NED position innovations (m/s, m)
    varInnov] ... % NED velocity and NED position innovation variance ((m/s)^2, m^2)
    = FuseVelPosNED( ...
    states, ... % predicted states from the INS (q0, ... , q3, VelN,E,D, PosN,E,D, WindN,E, P0, camera roll pitch yaw misalignment)
    P, ... % predicted covariance
    accNavMag, ... % magnitude of rate of change of velocity in navigation frame (m/s^2)
    FuseVelData, ... % Boolean to initiate fusion of velocity measurements
    VelNED, ... % NED velocity measurements (m/s)
    StatesAtVelTime, ... % States captured at GPs measurement time
    FusePosData,  ... % Boolean to initiate fusion of position measurements
    PosNE, ... % NE position measurements (m)
    StatesAtPosTime, ... % States captured at GPs measurement time
    FuseHgtData, ... % Boolean to initiate fusion of height measurements
    HgtMea, ... % D position measurement (m)
    StatesAtHgtTime, ... % States captured at height measurement time
    useAirspeed) % Boolean to indicate that an airspeed sensor is being used

% define persistent variables
persistent velFailCount;
if isempty(velFailCount)
    velFailCount = uint32(0);
end
persistent posFailCount;
if isempty(posFailCount)
    posFailCount = uint32(0);
end
persistent hgtFailCount;
if isempty(hgtFailCount)
    hgtFailCount = uint32(0);
end

% initialise measurement health flags to false
velHealth = 0;
posHealth = 0;
hgtHealth = 0;

% Specify GPS velocity induced error
velErr = single(0.15*accNavMag);
posErr = single(0.15*accNavMag);
% Specify the GPS and height measurement variances.
R_OBS = single([(0.1^2 + velErr^2) (0.1^2 + velErr^2) (0.1^2 + velErr^2) (2.0^2 + posErr^2) (2.0^2 + posErr^2) 2.0^2]);

% Specify the count before forcing use of GPS or height data after invalid
% data. We need to force GPS again sooner without
% airspeed data as the nav velocities will be unconstrained.
gpsRetryTime = single(30);
gpsRetryTimeNoTAS = single(5);
hgtRetryTime = single(30);
dt = single(0.02);
if useAirspeed
    maxVelFailCount = round(gpsRetryTime/dt);
    maxPosFailCount = maxVelFailCount;
else
    maxVelFailCount = round(gpsRetryTimeNoTAS/dt);
    maxPosFailCount = maxVelFailCount;
end
maxHgtFailCount = round(hgtRetryTime/dt);

% initialise the innovation vector
innovation = single(zeros(6,1));

% initialise the innovation variance vector
varInnov = single(zeros(6,1));

% Define the observation vector
observation = single([VelNED;PosNE;-HgtMea]);

% Perform sequential fusion of GPS and height measurements. This assumes that the
% errors in the dfferent velocity and position componenets are
% uncorrelated which is not true, however in the absence of covariance
% data from the GPS receiver it is the only assumption we can make
% so we might as well take advantage of the computational efficiencies
% associated with sequential fusion
if (FuseVelData || FusePosData || FuseHgtData)
    % calculate innovation variances
    for obsIndex = 1:6
        stateIndex = 4 + obsIndex;
        varInnov(obsIndex) = P(stateIndex,stateIndex) + R_OBS(obsIndex);
    end
    % calculate innovations and check validity against limits
    if FuseVelData
        velInnov = StatesAtVelTime(5:7) - VelNED;
        if (velInnov(1)*velInnov(1) + velInnov(2)*velInnov(2) + velInnov(3)*velInnov(3)) < 25.0*(varInnov(1) + varInnov(2) + varInnov(3)) || ...
                (velFailCount > maxVelFailCount)
            velHealth = 1;
            velFailCount = uint32(0);
        else
            velHealth = 0;
            velFailCount = velFailCount + uint32(1);
        end
    end
    if FusePosData
        posInnov = StatesAtPosTime(8:9) - PosNE;
        if (posInnov(1)*posInnov(1) + posInnov(2)*posInnov(2)) < 100.0*(varInnov(4) + varInnov(5)) || ...
                (posFailCount > maxPosFailCount)
            posHealth = 1;
            posFailCount = uint32(0);
        else
            posHealth = 0;
            posFailCount = posFailCount + uint32(1);
        end
    end
    if FusePosData
        hgtInnov = StatesAtHgtTime(10) + HgtMea;
        if (hgtInnov*hgtInnov) < 25.0*varInnov(6) || ...
                (hgtFailCount > maxHgtFailCount)
            hgtHealth = 1;
            hgtFailCount = uint32(0);
        else
            hgtHealth = 0;
            hgtFailCount = hgtFailCount + uint32(1);
        end
    end
    % Set range for sequential fusion of velocity and position measurements
    fuseData = zeros(1,6);
    if FuseVelData
        fuseData(1) = 1;
        fuseData(2) = 1;
        fuseData(3) = 1;
    end
    if FusePosData
        fuseData(4) = 1;
        fuseData(5) = 1;
    end
    if FuseHgtData
        fuseData(6) = 1;
    end
    % Fuse measurements sequentially
    for obsIndex = 1:6
        if fuseData(obsIndex)
            % Apply data health checks
            % If no airspeed data, start using GPS data after x seconds
            if (velHealth && (obsIndex >= 1 && obsIndex <= 3)) || ...
                    (posHealth && (obsIndex == 4 || obsIndex == 5)) || ...
                    (hgtHealth && (obsIndex == 6))
                stateIndex = 4 + obsIndex;
                % Calculate the measurement innovation, using states from the
                % appropriate time coordinate
                if (obsIndex >= 1 && obsIndex <= 3)
                    innovation(obsIndex) = StatesAtVelTime(stateIndex) - observation(obsIndex);
                elseif (obsIndex == 4 || obsIndex == 5)
                    innovation(obsIndex) = StatesAtPosTime(stateIndex) - observation(obsIndex);
                elseif (obsIndex == 6)
                    innovation(obsIndex) = StatesAtHgtTime(stateIndex) - observation(obsIndex);
                else
                    innovation(obsIndex) = 0.0;
                end
                
                % Calculate the Kalman Gain
                varInnov(obsIndex) = P(stateIndex,stateIndex) + R_OBS(obsIndex); % data logging only
                SK = 1/varInnov(obsIndex);
                K = P(:,stateIndex)*SK;
                % Calculate state corrections
                xk = K * innovation(obsIndex);
                % Update the covariance - take advantage of direct observation of a
                % single state at stateIndex
                %P = (I - K*H)*P;
                KHP = single(zeros(24,24));
                for rowIndex = 1:24
                    for colIndex = 1:24
                        KHP(rowIndex,colIndex) = K(rowIndex)*P(stateIndex,colIndex);
                    end
                end
                P = P - KHP;
                % Apply the state corrections and re-normaliase the quaternions
                states = states - xk;
                % Normalise the quaternion states
                quatMag = sqrt(states(1)^2 + states(2)^2 + states(3)^2 + states(4)^2);
                if (quatMag > 1e-12)
                    states(1:4) = states(1:4) / quatMag;
                end
            end
        end
    end
end
% Output covariance matrix and state vector
nextP = P;
nextStates = states;
end
